simulink model "colors"  (R2014a)
settings: Solver=FixedStepDiscrete  StartTime=0.0  StopTime=Inf  RelTol=1e-3
undefined symbols (not defined in the file): gray, Rec, SDTV
libraries: visionconversions x1, simulink x1, dspvision x1, visionsinks x1
settings Model: Creator=eruffaldi  LastModifiedBy=eruffaldi

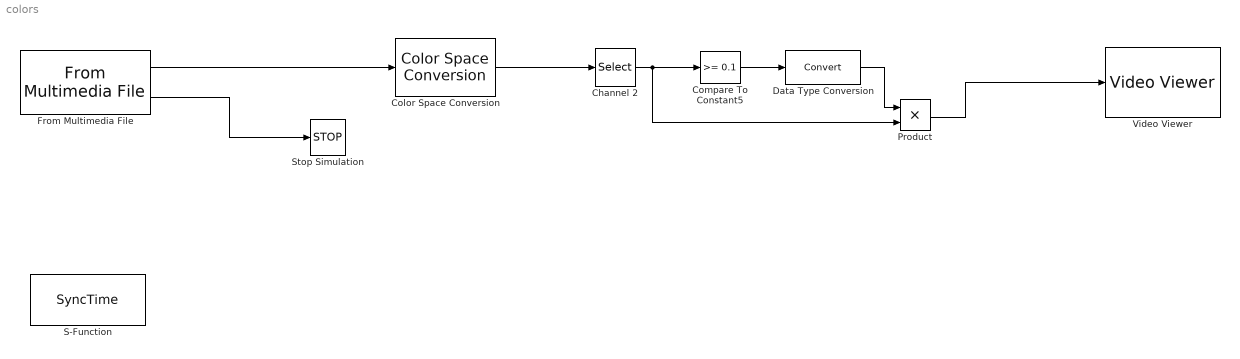
== system colors ==
  Channel 2 : Selector  NumberOfDimensions=3  InputPortWidth=3  IndexOptions=Select all,Select all,Index vector (dialog)  Indices=[1 3],1,[2]  OutputSizes=1,1,1
  Color Space Conversion : visionconversions/Color Space  Conversion  conversion=Obsolete  conversionActive=R'G'B' to Y'CbCr  wp_str=D65  rec=Rec. 601 (SDTV)  sys=1125/60/2:1  imagePorts=One multidimensional signal
  Compare To Constant5 : simulink/Logic and Bit Operations/Compare To Constant  relop=>=  const=0.1  OutDataTypeStr=boolean  ZeroCross=off
  Data Type Conversion : DataTypeConversion
  From Multimedia File : dspvision/From Multimedia File  inputFilename=viptrain.avi  loop=on  numPlays=inf  outputStreams=Video only  videoDataType=single  audioDataType=int16  inheritSampleTime=on  userDefinedSampleTime=1/30  noAudioOutput=off  isIntensityVideo=off  fourcc=RGB  colorVideoFormat=One multidimensional signal  outputEOF=on  dataOrg=Column-major  audioFrameSize=1024  computeAudioFrameSize=off  outSamplingMode=Frame based
  Product : Product
  S-Function : S-Function  Priority=1024  FunctionName=SyncTime  Parameters=dt  EnableBusSupport=off  mask{dt=1/30}
      mask prompts: dt "Period (s) or 0 for sleepless"
      mask Display:
      | port_label('output',1,'Unix Epoch s');
      | port_label('output',2,'Slept s');
  Stop Simulation : Stop
  Video Viewer : visionsinks/Video Viewer  inputType=Obsolete7b  imagePorts=One multidimensional signal  useColorMap=off  colormapValue=gray(256)  specRange=off  minInputVal=0  maxInputVal=255  FigPos=[681 700 410 300]  AxisZoom=on  trueSizedOnce=off  OpenAtMdlStart=on  DefaultConfigurationName=vipscopes.VideoViewerScopeCfg
  wires:
  From Multimedia File/2 -> Stop Simulation/1
  From Multimedia File/1 -> Color Space Conversion/1
  Color Space Conversion/1 -> Channel 2/1
  Channel 2/1 -> Product/2, Compare To Constant5/1
  Compare To Constant5/1 -> Data Type Conversion/1
  Data Type Conversion/1 -> Product/1
  Product/1 -> Video Viewer/1
